simulink model "test_PI_formation_gazebo_aerospace23a"  (R2023a)
settings: Solver=FixedStepAuto  StartTime=0.0  StopTime=inf  RelTol=1e-3
undefined symbols (not defined in the file or in its folder): angular, DiscIntNeverNeededParam, linear
libraries: ros2lib x11, simulink x4, robotcorelib x4
(part 2 of 2)

== matlab function test_PI_formation_gazebo_aerospace23a/MATLAB Function4 ==
  data: t input; D output
function D = fcn(t)

if t <= 40
    d1 = 0 ;
    d2 = 0;
    d3 = 0;
elseif t <= 75
    d1 = 0.5 + 0.2*sin(0.4*t)*0.5*cos(0.1*t) ;
    d2 = 0.5 + 0.1*cos(0.2*t);
    d3 = 0; %0.01;%*sin(0.1*t);
elseif t <= 110
    d1 = 0.65 + 0.1*sin(0.4*t)*0.5*cos(0.1*t) ; %2.2
    d2 = 0.75 + 0.05*cos(0.4*t)*0.5*cos(0.1*t);
    d3 = 0; %0.01;%*sin(0.1*t);
else
    d1 = 0.5 + 0.2*sin(0.4*t)*0.5*cos(0.1*t) ;
    d2 = 0.6 + 0.25*cos(0.4*t)*0.5*cos(0.1*t);
    d3 = 0; %0.01;%*sin(0.1*t);
end

D = [d1;d2;d3];  %[cos(yaw(1)) -sin(yaw(1)) 0;sin(yaw(1)) cos(yaw(1)) 0;0 0 1]*

== matlab function test_PI_formation_gazebo_aerospace23a/MATLAB Function1 ==
  data: sec input; gaz_time output; nanosec input
function gaz_time = fcn(sec, nanosec)

nanosec1 = double(nanosec)/1000000000; %*10^(-9);

sec1 = double(sec);

gaz_time = sec1 + nanosec1;
